simulink model "H_inf_discreto"  (R2024a)
settings: Solver=VariableStepAuto  StartTime=0.0  StopTime=50  RelTol=1e-3
undefined symbols (not defined in the file or in its folder): A_d, B_d, C_d, h_inf_discreto, T_s
libraries: simulink x1
settings Model: Creator=Luis Enrique Carmona  LastModifiedBy=Luis Enrique Carmona

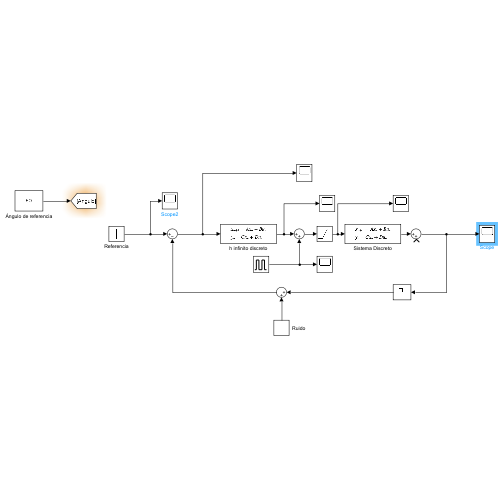
[thumbnail: Simulink's stored preview of the top-level diagram]
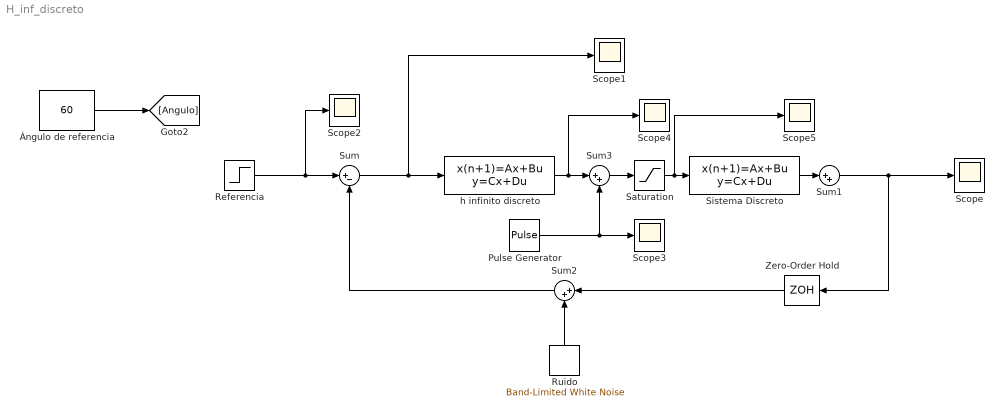
== system H_inf_discreto ==
  Pulse Generator : DiscretePulseGenerator  PulseType=Time based  Period=22  PulseWidth=5  PhaseDelay=1
  Referencia : Step  Time=0  After=50  SampleTime=0
  Ruido : simulink/Sources/Band-Limited White Noise  Cov=[0.1]  Ts=0.01  seed=[23341]
  Saturation : Saturate  UpperLimit=100  LowerLimit=0
  Scope{,1..5} (6 alike) : Scope
  Sistema Discreto : DiscreteStateSpace  A=A_d  B=B_d  C=C_d  D=0  SampleTime=T_s
  Sum : Sum  Inputs=|+-
  Sum1 : Sum  Inputs=|++
  Sum2 : Sum  Inputs=|++
  Sum3 : Sum  Inputs=|++
  Zero-Order Hold : ZeroOrderHold  SampleTime=0.01
  h infinito discreto : DiscreteStateSpace  A=h_inf_discreto.A  B=h_inf_discreto.B  C=h_inf_discreto.C  D=0  SampleTime=T_s
  Ángulo de referencia : Constant  Value=60
  wires:
  Sistema Discreto/1 -> Sum1/1
  h infinito discreto/1 -> Scope4/1, Sum3/1
  Sum2/1 -> Sum/2
  Referencia/1 -> Scope2/1, Sum/1
  Sum1/1 -> Zero-Order Hold/1, Scope/1
  Sum3/1 -> Saturation/1
  Zero-Order Hold/1 -> Sum2/1
  Sum/1 -> Scope1/1, h infinito discreto/1
  Pulse Generator/1 -> Sum3/2, Scope3/1
  Ángulo de referencia/1 -> [Angulo]
  Saturation/1 -> Scope5/1, Sistema Discreto/1
  Ruido/1 -> Sum2/2
